simulink model "AFMss_fp_obshas_uk"  (R2016b)
settings: Solver=ode4  StartTime=0.0  StopTime=trun  FixedStep=Ts  RelTol=1e-5  EnableMultiTasking=on
PreLoadFcn:
  | VSS_CONTROL_MODE=1;
  | VSS_LINEAR_CONTROL=Simulink.Variant('VSS_CONTROL_MODE==1');
  | VSS_MPC_CONTROL=Simulink.Variant('VSS_CONTROL_MODE == 2');
  | 
  | 
  | VSS_STATE_DIRECT=Simulink.Variant('VSS_STATE_MODE==1');
  | VSS_STATE_OBS=Simulink.Variant('VSS_STATE_MODE==2');
  | VSS_STATE_DIST_OBS=Simulink.Variant('VSS_STATE_MODE==3');
  | VSS_STATE_MODE=1;
undefined symbols (not defined in the file): C_ydist, Ident_obs, K_lqr, PLANT, r, rp, sim_obj, Ts, uss_0, w, wp, x0
libraries: cstblocks x2
settings Model: Creator=arnold  LastModifiedBy=arnold
settings DataIOCC: SaveFormat=Array  SaveOutput=off  SaveState=on  InspectSignalLogs=on  TimeSaveName=tout_ptos
settings OptimizationCC: LifeSpan=inf
settings DebuggingCC: SolverPrmCheckMsg=warning  SFUnexpectedBacktrackingDiag=warning  SFNoUnconditionalDefaultTransitionDiag=warning  SFExecutionAtInitializationDiag=none
settings HardwareCC: ProdBitPerPointer=32  ProdBitPerSizeT=32  ProdBitPerPtrDiffT=32  ProdLargestAtomicFloat=None  ProdIntDivRoundTo=Undefined  ProdEndianess=Unspecified  ProdWordSize=32  ProdHWDeviceType=32-bit Generic
settings ModelReferenceCC: PropagateSignalLabelsOutOfModel=off
settings GRTTargetCC: TargetLangStandard=C89/C90 (ANSI)  GeneratePreprocessorConditionals=Disable all
settings ConfigComp: CovMetricSettings=dw  CovHtmlReporting=on  CovSaveCumulativeToWorkspaceVar=on  CovSaveSingleToWorkspaceVar=on  CovExternalEMLEnable=off  CovSFcnEnable=off

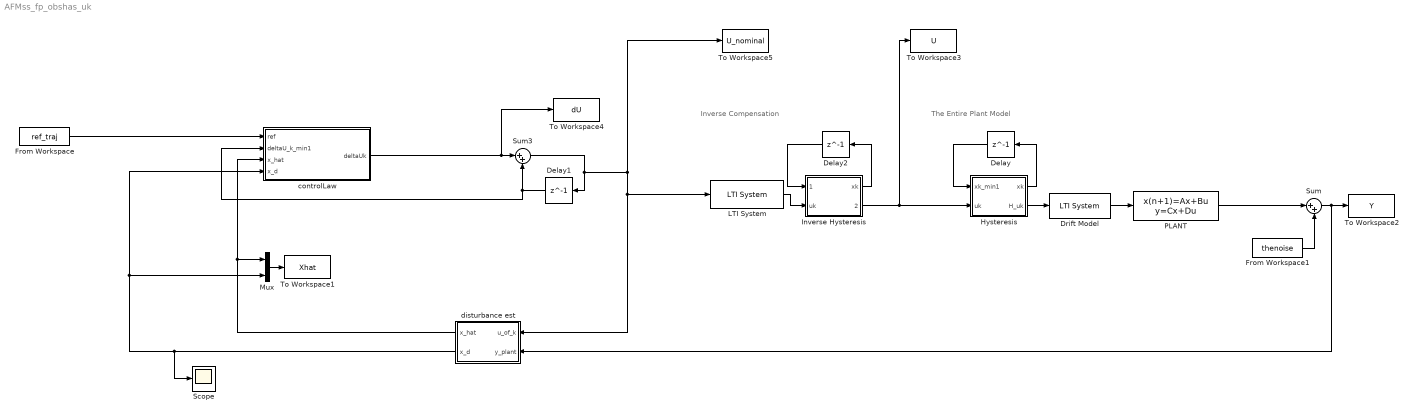
== system AFMss_fp_obshas_uk ==
  note: Inverse Compensation
  note: The Entire Plant Model
  Delay : Delay  DelayLength=1  InitialCondition=zeros(length(r),1)
  Delay1 : Delay  DelayLength=1  InitialCondition=uss_0  SampleTime=Ts
  Delay2 : Delay  DelayLength=1  InitialCondition=zeros(length(rp),1)
  Drift Model : cstblocks/LTI System  sys=sim_obj.gdrift  IC=x0_full
  From Workspace : FromWorkspace  VariableName=ref_traj  SampleTime=Ts
  From Workspace1 : FromWorkspace  VariableName=thenoise  SampleTime=Ts
  Hysteresis : MATLAB Function  TreatAsAtomicUnit=on
  Inverse Hysteresis : MATLAB Function  TreatAsAtomicUnit=on
  LTI System : cstblocks/LTI System  sys=sim_obj.gdrift_inv  IC=[]
  Mux : Mux  Inputs=2
  PLANT : DiscreteStateSpace  A=PLANT.a  B=PLANT.b  C=PLANT.c  D=zeros(size(PLANT.c,1),1)  X0=x0  SampleTime=Ts
  Scope : Scope
  Sum : Sum  Inputs=|++
  Sum3 : Sum  Inputs=|++
  To Workspace1 : ToWorkspace  VariableName=Xhat  SaveFormat=Timeseries  SampleTime=-1
      settings: Save2DSignal=2-D array (concatenate along first dimension)
  To Workspace2 : ToWorkspace  VariableName=Y  SaveFormat=Timeseries  SampleTime=-1
      settings: Save2DSignal=2-D array (concatenate along first dimension)
  To Workspace3 : ToWorkspace  VariableName=U  SaveFormat=Timeseries  SampleTime=-1
      settings: Save2DSignal=2-D array (concatenate along first dimension)
  To Workspace4 : ToWorkspace  VariableName=dU  SaveFormat=Timeseries  SampleTime=-1
      settings: Save2DSignal=2-D array (concatenate along first dimension)
  To Workspace5 : ToWorkspace  VariableName=U_nominal  SaveFormat=Timeseries  SampleTime=-1
      settings: Save2DSignal=2-D array (concatenate along first dimension)
  controlLaw : Subsystem
  disturbance est : Subsystem  VariantControl=VSS_STATE_DIST_OBS
  wires:
  Sum/1 -> disturbance est/2(y_plant), To Workspace2/1
  disturbance est/1(x_hat) -> Mux/1, controlLaw/3(x_hat)
  From Workspace1/1 -> Sum/2
  PLANT/1 -> Sum/1
  Delay1/1 -> Sum3/2, controlLaw/2(deltaU_k_min1)
  Drift Model/1 -> PLANT/1
  Sum3/1 -> To Workspace5/1, LTI System/1, disturbance est/1(u_of_k), Delay1/1
  controlLaw/1(deltaUk) -> To Workspace4/1, Sum3/1
  From Workspace/1 -> controlLaw/1(ref)
  disturbance est/2(x_d) -> Scope/1, Mux/2, controlLaw/4(x_d)
  Hysteresis/2(H_uk) -> Drift Model/1
  Hysteresis/1(xk) -> Delay/1
  Delay/1 -> Hysteresis/1(xk_min1)
  LTI System/1 -> Inverse Hysteresis/2(uk)
  Inverse Hysteresis/2(H_inv_uk) -> To Workspace3/1, Hysteresis/2(uk)
  Inverse Hysteresis/1(xk) -> Delay2/1
  Delay2/1 -> Inverse Hysteresis/1(xk_min1)
  Mux/1 -> To Workspace1/1

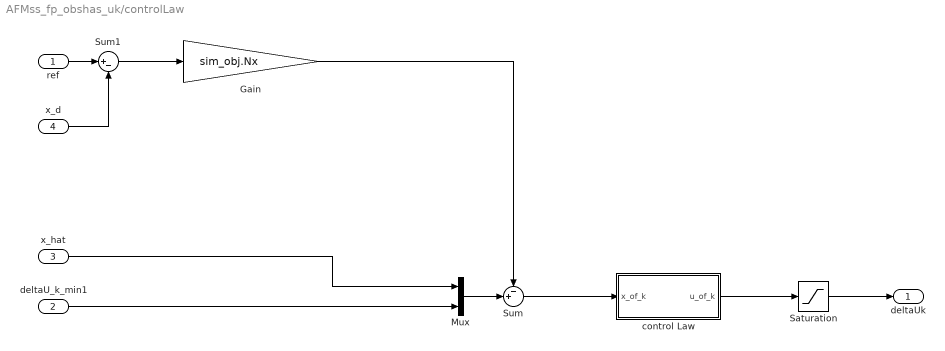
== system AFMss_fp_obshas_uk/controlLaw ==
  ref : Inport
  deltaU_k_min1 : Inport  Port=2
  x_hat : Inport  Port=3
  x_d : Inport  Port=4
  Gain : Gain  Gain=sim_obj.Nx
  Mux : Mux  Inputs=2
  Saturation : Saturate  UpperLimit=sim_obj.du_max  LowerLimit=-sim_obj.du_max
  Sum : Sum  Inputs=-+|
  Sum1 : Sum  Inputs=|+-
  control Law : Subsystem  Variant=on
  deltaUk : Outport
  wires:
  Saturation/1 -> deltaUk/1
  control Law/1(u_of_k) -> Saturation/1
  ref/1 -> Sum1/1
  Sum/1 -> control Law/1(x_of_k)
  x_hat/1 -> Mux/1
  deltaU_k_min1/1 -> Mux/2
  Mux/1 -> Sum/2
  Gain/1 -> Sum/1
  Sum1/1 -> Gain/1
  x_d/1 -> Sum1/2

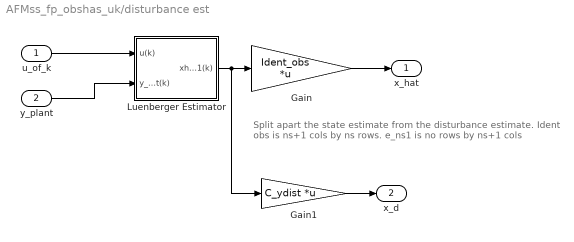
== system AFMss_fp_obshas_uk/disturbance est ==
  note: Split apart the state estimate from the disturbance estimate.
      | Ident obs is ns+1 cols by ns rows. e_ns1 is no rows by ns+1 cols
  u_of_k : Inport
  y_plant : Inport  Port=2
  Gain : Gain  Gain=Ident_obs  Multiplication=Matrix(K*u)
  Gain1 : Gain  Gain=C_ydist  Multiplication=Matrix(K*u)
  Luenberger Estimator : Subsystem  AncestorBlock=customLibFcns/Input Delay Luenberger Estimator
  x_hat : Outport
  x_d : Outport  Port=2
  wires:
  u_of_k/1 -> Luenberger Estimator/1(u(k))
  Luenberger Estimator/1(xhat_1(k)) -> Gain1/1, Gain/1
  y_plant/1 -> Luenberger Estimator/2(y_plant(k))
  Gain/1 -> x_hat/1
  Gain1/1 -> x_d/1

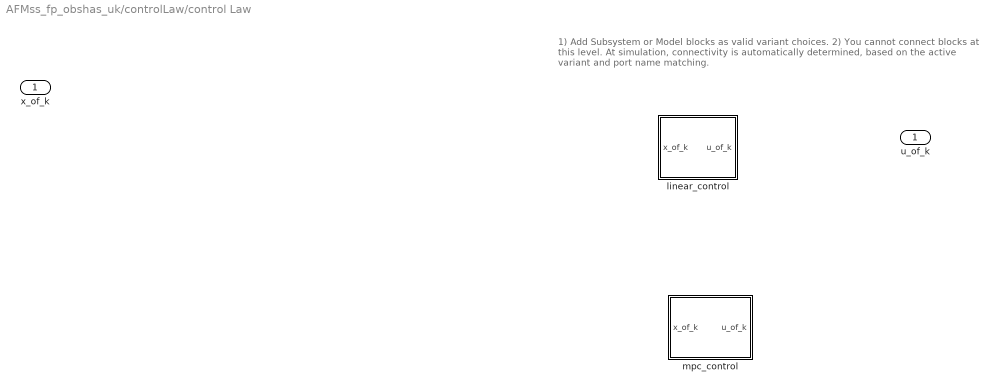
== system AFMss_fp_obshas_uk/controlLaw/control Law ==
  note: 1) Add Subsystem or Model blocks as valid variant choices.
      | 2) You cannot connect blocks at this level. At simulation, connectivity is automatically
      | determined, based on the active variant and port name matching.
  x_of_k : Inport
  linear_control : Subsystem  VariantControl=VSS_LINEAR_CONTROL
  mpc_control : Subsystem  VariantControl=VSS_MPC_CONTROL
  u_of_k : Outport

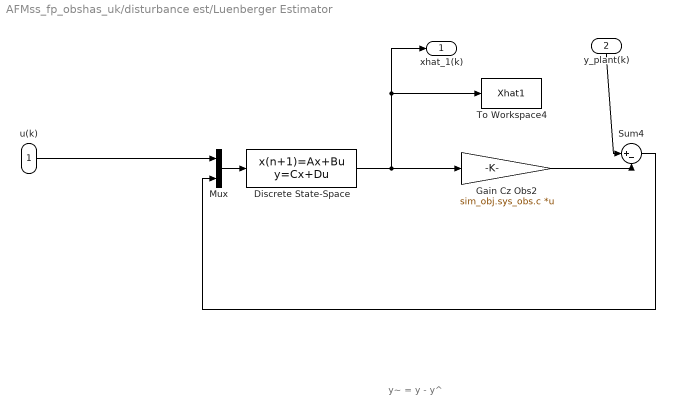
== system AFMss_fp_obshas_uk/disturbance est/Luenberger Estimator ==
  note: y~ = y - y^
  u(k) : Inport
  y_plant(k) : Inport  Port=2
  Discrete State-Space : DiscreteStateSpace  A=sim_obj.sys_obs.a  B=[sim_obj.sys_obs.b, sim_obj.L]  C=eye(length(sim_obj.sys_obs.b))  D=zeros(length(sim_obj.sys_obs.b), 2)  X0=sim_obj.x0_obs  SampleTime=Ts
  Gain Cz Obs2 : Gain  Gain=sim_obj.sys_obs.c  Multiplication=Matrix(K*u)
  Mux : Mux  Inputs=2
  Sum4 : Sum  Inputs=|+-
  To Workspace4 : ToWorkspace  VariableName=Xhat1  SaveFormat=Timeseries  SampleTime=-1
      settings: Save2DSignal=2-D array (concatenate along first dimension)
  xhat_1(k) : Outport
  wires:
  Sum4/1 -> Mux/2
  u(k)/1 -> Mux/1
  Mux/1 -> Discrete State-Space/1
  Discrete State-Space/1 -> Gain Cz Obs2/1, To Workspace4/1, xhat_1(k)/1
  Gain Cz Obs2/1 -> Sum4/2
  y_plant(k)/1 -> Sum4/1

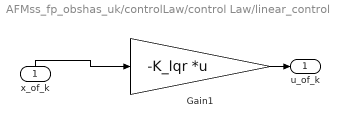
== system AFMss_fp_obshas_uk/controlLaw/control Law/linear_control ==
  x_of_k : Inport
  Gain1 : Gain  Gain=-K_lqr  Multiplication=Matrix(K*u)
  u_of_k : Outport
  wires:
  x_of_k/1 -> Gain1/1
  Gain1/1 -> u_of_k/1

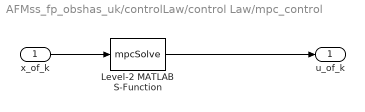
== system AFMss_fp_obshas_uk/controlLaw/control Law/mpc_control ==
  x_of_k : Inport
  Level-2 MATLAB S-Function : M-S-Function  FunctionName=mpcSolve  Parameters=mpcProb
  u_of_k : Outport
  wires:
  x_of_k/1 -> Level-2 MATLAB S-Function/1
  Level-2 MATLAB S-Function/1 -> u_of_k/1

== matlab function AFMss_fp_obshas_uk/Inverse Hysteresis ==
  data: xk output; xk_min1 input; uk input; H_inv_uk output; rp parameter; wp parameter
function [xk, H_inv_uk] = fcn(xk_min1, uk, rp, wp)
  % Implement simple IP hysteresis model.
  if length(rp) > 1
    xk = rp(:)*0;
    for j = 1:length(rp)
      xk(j) = max(uk - rp(j), min(uk+rp(j), xk_min1(j)));
    end
    
    H_inv_uk = wp'*xk(:);
  else
    xk = xk_min1;
    H_inv_uk = uk;
  end
end

== matlab function AFMss_fp_obshas_uk/Hysteresis ==
  data: xk output; xk_min1 input; uk input; H_uk output; r parameter; w parameter
function [xk, H_uk] = fcn(xk_min1, uk, r, w)
  % Implement simple IP hysteresis model.
  if length(r) > 1
    xk = r(:)*0;
    for j = 1:length(r)
      xk(j) = max(uk - r(j), min(uk+r(j), xk_min1(j)));
    end
    
    H_uk = w'*xk(:);
  else
    xk = xk_min1;
    H_uk = uk;
  end
end
